simulink subsystem "Day1_Scenario_1"  (R2024a)
settings: Solver=VariableStepAuto  StartTime=0.0  StopTime=10.0  RelTol=1e-3
libraries: CarMaker4SL x1
settings Model: Creator=junhyung.cha  LastModifiedBy=User

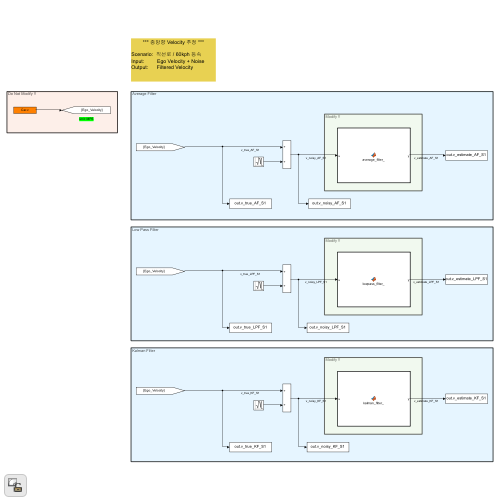
[thumbnail: Simulink's stored preview of the top-level diagram]
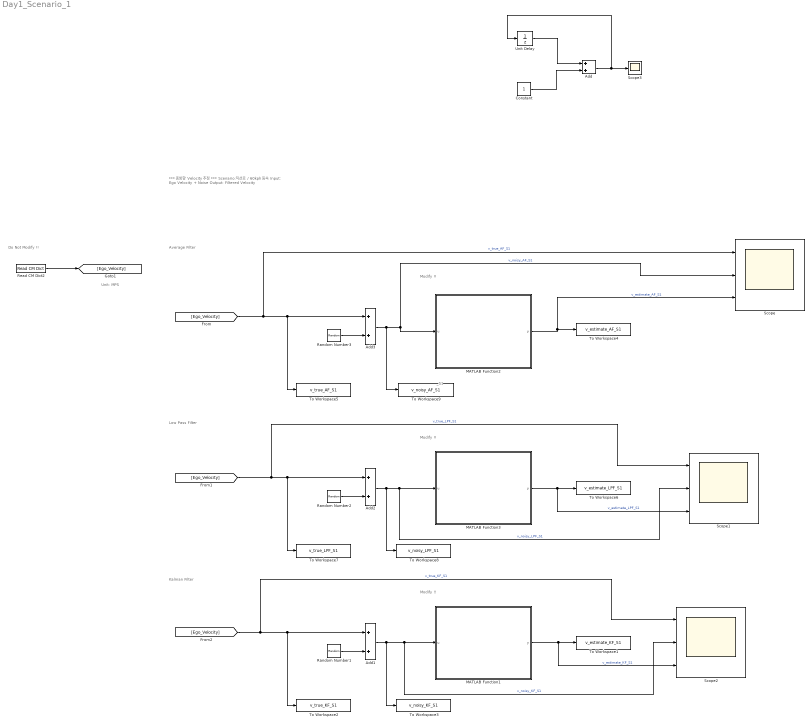
== system Day1_Scenario_1 ==
  note: _S1
  note: Modify !!
  note: Modify !!
  note: Modify !!
  note: Average Filter
  note: Low Pass Filter
  note: Kalman Filter
  note: *** 종방향 Velocity 추정 ***
      |
      | Scenario: 직선로 / 60kph 등속
      | Input: Ego Velocity + Noise
      | Output: Filtered Velocity
  note: Do Not Modify !!
  note: Unit: MPS
  Add{,1..3} (4 alike) : Sum
  Constant : Constant
  MATLAB Function1 : MATLAB Function  TreatAsAtomicUnit=on
  MATLAB Function2 : MATLAB Function  TreatAsAtomicUnit=on
  MATLAB Function3 : MATLAB Function  TreatAsAtomicUnit=on
  Random Number1 : RandomNumber
  Random Number2 : RandomNumber
  Random Number3 : RandomNumber
  Read CM Dict2 : CarMaker4SL/Read CM Dict  xname=Car.v  xsync=off  xstime=Inherited
  Scope : Scope  NumInputPorts=3
  Scope1 : Scope  NumInputPorts=3
  Scope2 : Scope  NumInputPorts=3
  Scope3 : Scope
  To Workspace1 : ToWorkspace  VariableName=v_estimate_KF_S1  SaveFormat=Timeseries  SampleTime=-1
  To Workspace2 : ToWorkspace  VariableName=v_true_KF_S1  SaveFormat=Timeseries  SampleTime=-1
  To Workspace3 : ToWorkspace  VariableName=v_noisy_KF_S1  SaveFormat=Timeseries  SampleTime=-1
  To Workspace4 : ToWorkspace  VariableName=v_estimate_AF_S1  SaveFormat=Timeseries  SampleTime=-1
  To Workspace5 : ToWorkspace  VariableName=v_true_AF_S1  SaveFormat=Timeseries  SampleTime=-1
  To Workspace6 : ToWorkspace  VariableName=v_estimate_LPF_S1  SaveFormat=Timeseries  SampleTime=-1
  To Workspace7 : ToWorkspace  VariableName=v_true_LPF_S1  SaveFormat=Timeseries  SampleTime=-1
  To Workspace8 : ToWorkspace  VariableName=v_noisy_LPF_S1  SaveFormat=Timeseries  SampleTime=-1
  To Workspace9 : ToWorkspace  VariableName=v_noisy_AF_S1  SaveFormat=Timeseries  SampleTime=-1
  Unit Delay : UnitDelay  InitialCondition=1  SampleTime=-1  HasFrameUpgradeWarning=on
  wires:
  Random Number2/1 -> Add2/2
  [Ego_Velocity] -> Add2/1, To Workspace7/1, Scope1/1  "v_true_LPF_S1"
  Add2/1 -> MATLAB Function3/1(u), Scope1/2, To Workspace8/1  "v_noisy_LPF_S1"
  MATLAB Function3/1(y) -> To Workspace6/1, Scope1/3  "v_estimate_LPF_S1"
  [Ego_Velocity] -> Add1/1, To Workspace2/1, Scope2/1  "v_true_KF_S1"
  MATLAB Function1/1(y) -> To Workspace1/1, Scope2/3  "v_estimate_KF_S1"
  Random Number1/1 -> Add1/2
  Add1/1 -> MATLAB Function1/1(u), Scope2/2, To Workspace3/1  "v_noisy_KF_S1"
  MATLAB Function2/1(y) -> To Workspace4/1, Scope/3  "v_estimate_AF_S1"
  Random Number3/1 -> Add3/2
  [Ego_Velocity] -> Scope/1, To Workspace5/1, Add3/1  "v_true_AF_S1"
  Add3/1 -> MATLAB Function2/1(u), Scope/2, To Workspace9/1  "v_noisy_AF_S1"
  Read CM Dict2/1 -> [Ego_Velocity]
  Constant/1 -> Add/2
  Unit Delay/1 -> Add/1
  Add/1 -> Scope3/1, Unit Delay/1

== matlab function Day1_Scenario_1/MATLAB Function1 ==
  settings: updateMethod=DISCRETE  sampleTime=0.05
  data: u input; y output
function y = kalman_filter_(u)
    persistent A B C D Q R x_estimate P_estimate input_u
    
    if isempty(x_estimate)
        step_time = 0.1;
        m = 0.1;
        modelVariance = 0.01;
        measureVariance = 1.0;
        errorVariance_init = 10.0;
        
        A = 1.0;
        B = step_time / m;
        C = 1.0;
        D = 0.0;
        Q = modelVariance;
        R = measureVariance;
        
        x_estimate = u;
        P_estimate = errorVariance_init;
        
        input_u = 0;   % <<== input_u를 내부에서 상수로 지정
    end
    
    % Prediction
    x_pred = A * x_estimate + B * input_u;
    P_pred = A * P_estimate * A + Q;
    
    % Kalman Gain
    K = P_pred * C / (C * P_pred * C + R);
    
    % Update
    x_estimate = x_pred + K * (u - C * x_pred);
    P_estimate = (1 - K * C) * P_pred;
    
    y = x_estimate;
end

== matlab function Day1_Scenario_1/MATLAB Function2 ==
  settings: updateMethod=DISCRETE  sampleTime=0.05
  data: u input; y output
function y = exponential_moving_average(u)
    persistent y_estimate k
    
    if isempty(y_estimate)
        y_estimate = u; % 초기값
        k = 1;
    else
        k = k + 1;
        y_estimate = ((k - 1) / k) * y_estimate + (1 / k) * u;
    end
    
    y = y_estimate;
end

== matlab function Day1_Scenario_1/MATLAB Function3 ==
  settings: updateMethod=DISCRETE  sampleTime=0.05
  data: u input; y output
function y = lowpass_filter_(u)
    persistent y_estimate alpha
    
    if isempty(y_estimate)
        alpha = 0.9;       % smoothing factor 초기값
        y_estimate = u;     % 첫 측정값 저장
    end
    
    y_estimate = alpha * y_estimate + (1 - alpha) * u;
    y = y_estimate;
end
